simulink subsystem "Choose_starTracker"  (R2022b)
settings: Solver=VariableStepAuto  StartTime=0.0  StopTime=10.0  RelTol=1e-3
undefined symbols (not defined in the file or in its folder): alfa1, alfa2, degtorad, environment, sat, sensors
libraries: vrlib x1
settings Model: Creator=brent  LastModifiedBy=Nicolò

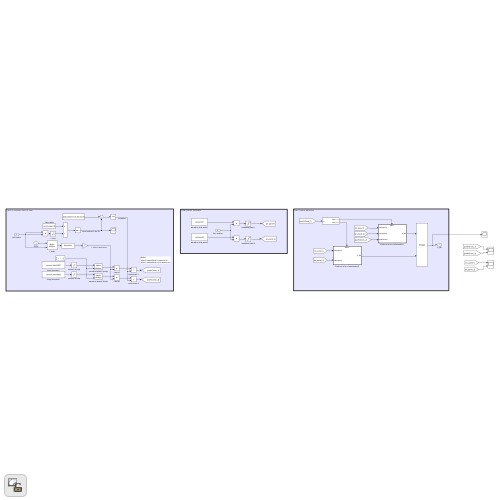
[thumbnail: Simulink's stored preview of the top-level diagram]
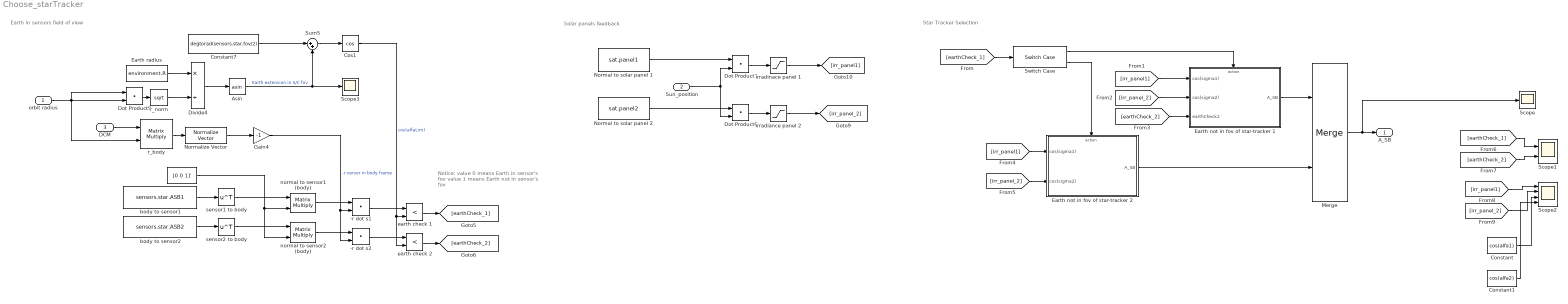
== system Choose_starTracker ==
  note: Notice:
      | value 0 means Earth in sensor's fov
      | value 1 means Earth not in sensor's fov
  note: Solar panels feedback
  note: Star Tracker Selection
  note: Earth in sensors field of view
  orbit radius : Inport
  Sun_position : Inport  Port=2
  DCM : Inport  Port=3
  " " : Constant  Value=[0 0 1]'
  -r dot s1 : DotProduct  OutDataTypeStr=Inherit: Inherit via internal rule
  -r dot s2 : DotProduct  OutDataTypeStr=Inherit: Inherit via internal rule
  Asin : Trigonometry  Operator=asin
  Constant : Constant  Value=cos(alfa1)
  Constant1 : Constant  Value=cos(alfa2)
  Constant7 : Constant  Value=degtorad(sensors.star.fov/2)
  Cos1 : Trigonometry  Operator=cos
  Divide4 : Product  Inputs=*/
  Dot Product6 : DotProduct  OutDataTypeStr=Inherit: Inherit via internal rule
  Dot Product7 : DotProduct  OutDataTypeStr=Inherit: Inherit via internal rule
  Dot Product9 : DotProduct  OutDataTypeStr=Inherit: Inherit via internal rule
  Earth not in fov of star-tracker 1 : Subsystem  TreatAsAtomicUnit=on
  Earth not in fov of star-tracker 2 : Subsystem  TreatAsAtomicUnit=on
  Earth radius : Constant  Value=environment.R
  Gain4 : Gain  Gain=-1
  Merge : Merge
  Normal to solar panel 1 : Constant  Value=sat.panel1
  Normal to solar panel 2 : Constant  Value=sat.panel2
  Normalize Vector : vrlib/Utilities/Normalize Vector  maxzero=0
  Scope : Scope
  Scope1 : Scope  NumInputPorts=2
  Scope2 : Scope  NumInputPorts=4
  Scope3 : Scope
  Sum5 : Sum  Inputs=|++
  Switch Case : SwitchCase  CaseConditions={1, 0}  ShowDefaultCase=off
  body to sensor1 : Constant  Value=sensors.star.ASB1
  body to sensor2 : Constant  Value=sensors.star.ASB2
  earth check 1 : RelationalOperator  Operator=<  OutDataTypeStr=fixdt(1,16)  RndMeth=Simplest  InputSameDT=off
  earth check 2 : RelationalOperator  Operator=<  OutDataTypeStr=fixdt(1,16)  RndMeth=Simplest  InputSameDT=off
  irradiance panel 2 : Saturate  UpperLimit=1  LowerLimit=0
  irradinace panel 1 : Saturate  UpperLimit=1  LowerLimit=0
  normal to sensor1 (body) : Product  Multiplication=Matrix(*)
  normal to sensor2 (body) : Product  Multiplication=Matrix(*)
  r_body : Product  Multiplication=Matrix(*)
  r_norm : Sqrt
  sensor1 to body : Math  Operator=transpose
  sensor2 to body : Math  Operator=transpose
  A_SB : Outport
  wires:
  sensor1 to body/1 -> normal to sensor1 (body)/1
  sensor2 to body/1 -> normal to sensor2 (body)/1
  earth check 1/1 -> [earthCheck_1]
  earth check 2/1 -> [earthCheck_2]
  DCM/1 -> r_body/1
  orbit radius/1 -> Dot Product9/1, r_body/2, Dot Product9/2
  normal to sensor2 (body)/1 -> -r dot s2/1
  Gain4/1 -> -r dot s1/2, -r dot s2/2  "-r versor in body frame"
  " "/1 -> normal to sensor1 (body)/2, normal to sensor2 (body)/2
  r_body/1 -> Normalize Vector/1
  -r dot s1/1 -> earth check 1/1
  body to sensor2/1 -> sensor2 to body/1
  Cos1/1 -> earth check 1/2, earth check 2/2  "cos(alfaLim)"
  body to sensor1/1 -> sensor1 to body/1
  Earth radius/1 -> Divide4/1
  Asin/1 -> Scope3/1, Sum5/2  "Earth extension in S/C fov"
  Dot Product9/1 -> r_norm/1
  -r dot s2/1 -> earth check 2/1
  normal to sensor1 (body)/1 -> -r dot s1/1
  Normalize Vector/1 -> Gain4/1
  r_norm/1 -> Divide4/2
  Sum5/1 -> Cos1/1
  Divide4/1 -> Asin/1
  Constant7/1 -> Sum5/1
  Dot Product7/1 -> irradinace panel 1/1
  Dot Product6/1 -> irradiance panel 2/1
  Normal to solar panel 2/1 -> Dot Product6/1
  irradiance panel 2/1 -> [irr_panel_2]
  irradinace panel 1/1 -> [irr_panel1]
  Sun_position/1 -> Dot Product7/2, Dot Product6/2
  Normal to solar panel 1/1 -> Dot Product7/1
  [earthCheck_1] -> Switch Case/1
  Switch Case/1 -> Earth not in fov of star-tracker 1/Action
  [irr_panel1] -> Earth not in fov of star-tracker 1/1(cos(sigma1))
  [irr_panel_2] -> Earth not in fov of star-tracker 1/2(cos(sigma2))
  [earthCheck_2] -> Earth not in fov of star-tracker 1/3(earthCheck2)
  [irr_panel1] -> Earth not in fov of star-tracker 2/1(cos(sigma1))
  [irr_panel_2] -> Earth not in fov of star-tracker 2/2(cos(sigma2))
  Earth not in fov of star-tracker 1/1(A_SB) -> Merge/1
  Earth not in fov of star-tracker 2/1(A_SB) -> Merge/2
  Merge/1 -> A_SB/1, Scope/1
  Switch Case/2 -> Earth not in fov of star-tracker 2/Action
  [earthCheck_1] -> Scope1/1
  [earthCheck_2] -> Scope1/2
  [irr_panel1] -> Scope2/1
  [irr_panel_2] -> Scope2/2
  Constant/1 -> Scope2/3
  Constant1/1 -> Scope2/4

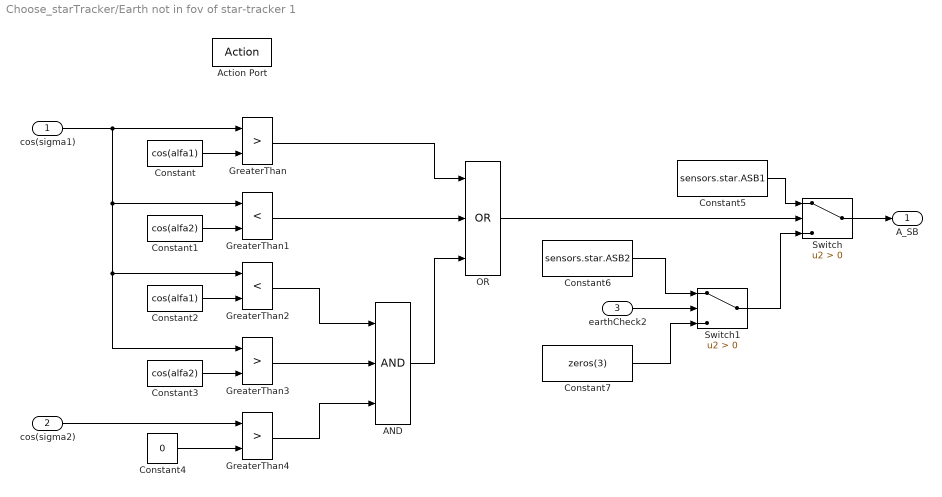
== system Choose_starTracker/Earth not in fov of star-tracker 1 ==
  cos(sigma1) : Inport
  cos(sigma2) : Inport  Port=2
  earthCheck2 : Inport  Port=3
  Action Port : ActionPort
  AND : Logic  Inputs=3  IconShape=distinctive  AllPortsSameDT=off  OutDataTypeStr=boolean
  Constant : Constant  Value=cos(alfa1)
  Constant1 : Constant  Value=cos(alfa2)
  Constant2 : Constant  Value=cos(alfa1)
  Constant3 : Constant  Value=cos(alfa2)
  Constant4 : Constant  Value=0
  Constant5 : Constant  Value=sensors.star.ASB1
  Constant6 : Constant  Value=sensors.star.ASB2
  Constant7 : Constant  Value=zeros(3)
  GreaterThan : RelationalOperator  Operator=>  OutDataTypeStr=boolean  RndMeth=Simplest  InputSameDT=off
  GreaterThan1 : RelationalOperator  Operator=<  OutDataTypeStr=boolean  RndMeth=Simplest  InputSameDT=off
  GreaterThan2 : RelationalOperator  Operator=<  OutDataTypeStr=boolean  RndMeth=Simplest  InputSameDT=off
  GreaterThan3 : RelationalOperator  Operator=>  OutDataTypeStr=boolean  RndMeth=Simplest  InputSameDT=off
  GreaterThan4 : RelationalOperator  Operator=>  OutDataTypeStr=boolean  RndMeth=Simplest  InputSameDT=off
  OR : Logic  Operator=OR  Inputs=3  IconShape=distinctive  AllPortsSameDT=off  OutDataTypeStr=fixdt(1,16)
  Switch : Switch  Criteria=u2 > Threshold  SaturateOnIntegerOverflow=off  InputSameDT=off
  Switch1 : Switch  Criteria=u2 > Threshold  SaturateOnIntegerOverflow=off  InputSameDT=off
  A_SB : Outport
  wires:
  Constant7/1 -> Switch1/3
  Constant6/1 -> Switch1/1
  Switch1/1 -> Switch/3
  Constant5/1 -> Switch/1
  Switch/1 -> A_SB/1
  earthCheck2/1 -> Switch1/2
  OR/1 -> Switch/2
  AND/1 -> OR/3
  GreaterThan1/1 -> OR/2
  GreaterThan/1 -> OR/1
  GreaterThan4/1 -> AND/3
  GreaterThan2/1 -> AND/1
  GreaterThan3/1 -> AND/2
  Constant4/1 -> GreaterThan4/2
  cos(sigma2)/1 -> GreaterThan4/1
  cos(sigma1)/1 -> GreaterThan/1, GreaterThan1/1, GreaterThan3/1, GreaterThan2/1
  Constant2/1 -> GreaterThan2/2
  Constant3/1 -> GreaterThan3/2
  Constant1/1 -> GreaterThan1/2
  Constant/1 -> GreaterThan/2

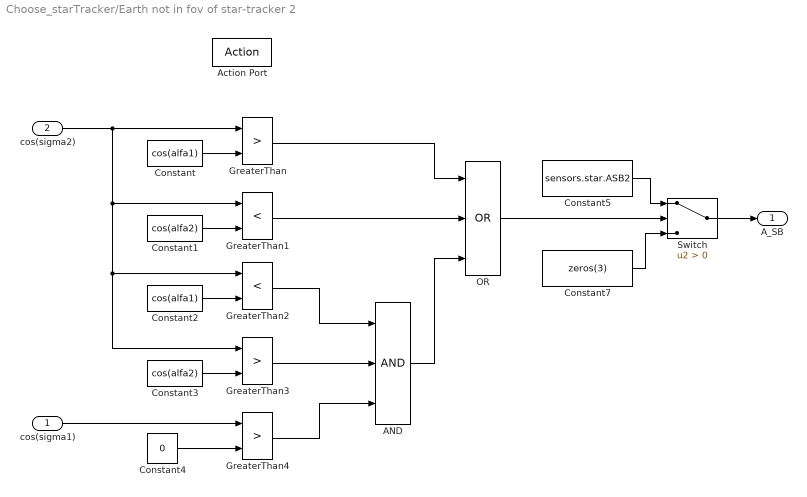
== system Choose_starTracker/Earth not in fov of star-tracker 2 ==
  cos(sigma1) : Inport
  cos(sigma2) : Inport  Port=2
  Action Port : ActionPort
  AND : Logic  Inputs=3  IconShape=distinctive  AllPortsSameDT=off  OutDataTypeStr=boolean
  Constant : Constant  Value=cos(alfa1)
  Constant1 : Constant  Value=cos(alfa2)
  Constant2 : Constant  Value=cos(alfa1)
  Constant3 : Constant  Value=cos(alfa2)
  Constant4 : Constant  Value=0
  Constant5 : Constant  Value=sensors.star.ASB2
  Constant7 : Constant  Value=zeros(3)
  GreaterThan : RelationalOperator  Operator=>  OutDataTypeStr=boolean  RndMeth=Simplest  InputSameDT=off
  GreaterThan1 : RelationalOperator  Operator=<  OutDataTypeStr=boolean  RndMeth=Simplest  InputSameDT=off
  GreaterThan2 : RelationalOperator  Operator=<  OutDataTypeStr=boolean  RndMeth=Simplest  InputSameDT=off
  GreaterThan3 : RelationalOperator  Operator=>  OutDataTypeStr=boolean  RndMeth=Simplest  InputSameDT=off
  GreaterThan4 : RelationalOperator  Operator=>  OutDataTypeStr=boolean  RndMeth=Simplest  InputSameDT=off
  OR : Logic  Operator=OR  Inputs=3  IconShape=distinctive  AllPortsSameDT=off  OutDataTypeStr=fixdt(1,16)
  Switch : Switch  Criteria=u2 > Threshold  SaturateOnIntegerOverflow=off  InputSameDT=off
  A_SB : Outport
  wires:
  Constant/1 -> GreaterThan/2
  Constant1/1 -> GreaterThan1/2
  Constant3/1 -> GreaterThan3/2
  Constant2/1 -> GreaterThan2/2
  cos(sigma2)/1 -> GreaterThan2/1, GreaterThan3/1, GreaterThan1/1, GreaterThan/1
  cos(sigma1)/1 -> GreaterThan4/1
  Constant4/1 -> GreaterThan4/2
  GreaterThan3/1 -> AND/2
  GreaterThan2/1 -> AND/1
  GreaterThan4/1 -> AND/3
  GreaterThan/1 -> OR/1
  GreaterThan1/1 -> OR/2
  AND/1 -> OR/3
  OR/1 -> Switch/2
  Switch/1 -> A_SB/1
  Constant5/1 -> Switch/1
  Constant7/1 -> Switch/3
